simulink model "Weiv_filter_V1_1"  (R2017b)
settings: Solver=ode4  StartTime=0.0  StopTime=5.9443  RelTol=1e-3
undefined symbols (not defined in the file or in its folder): dfilt, get
libraries: dspobslib x2, dspvision x1, dspsnks4 x1
settings Model: Creator=root  LastModifiedBy=root

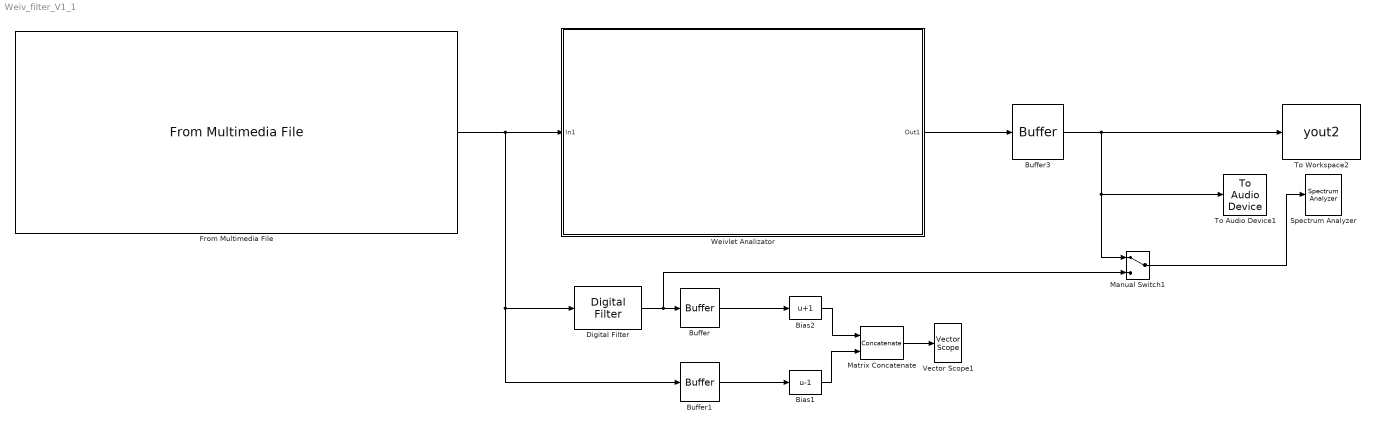
== system Weiv_filter_V1_1 ==
  Bias1 : Bias  Bias=-1
  Bias2 : Bias  Bias=1
  Buffer : Buffer  N=441
  Buffer1 : Buffer  N=441
  Buffer3 : Buffer  N=512
  Digital Filter : dspobslib/Digital Filter  TypePopup=IIR (poles & zeros)  IIRFiltStruct=Direct form II transposed  AllPoleFiltStruct=Direct form  FIRFiltStruct=Direct form  CoeffSource=Specify via dialog  NumCoeffs=[0 0.0554]  DenCoeffs=[1 -0.9446]  BiQuadCoeffs=[1 0.3 0.4 1 0.1 0.2]  LatticeCoeffs=[0.2 0.4]  denIgnore=on  FiltPerSampPopup=One filter per frame  IC=0  ICnum=0  ICden=0  roundingMode=Floor  overflowMode=off  ScaleValues=1  scaleValueFracLength=14  stageInFracLength=15  stageOutFracLength=15  FilterSource=Specify via dialog  dfiltObjectName=dfilt.dffir([1 2 1])  InputProcessing=Inherited (this choice will be removed - see release notes)
      settings: SourceProductName=DSP System Toolbox  SourceProductBaseCode=DS
  From Multimedia File : dspvision/From Multimedia File  inputFilename=/mnt/work/develop/matlab/voip/source/58691/MyTest.wav  loop=on  numPlays=inf  outputStreams=Audio only  videoDataType=single  audioDataType=double  inheritSampleTime=on  userDefinedSampleTime=1/30  noAudioOutput=off  isIntensityVideo=off  fourcc=RGB  colorVideoFormat=Separate color signals  outputEOF=off  dataOrg=Column-major  audioFrameSize=512  computeAudioFrameSize=off  outSamplingMode=Frame based
      settings: SourceProductBaseCode=VP
  Manual Switch1 : ManualSwitch
  Matrix Concatenate : Concatenate  Mode=Multidimensional array  ConcatenateDimension=2
  Spectrum Analyzer : SpectrumAnalyzer
  To Audio Device1 : dspobslib/To Audio Device  deviceName=Default  inheritSampleRate=on  sampleRate=44100  deviceDatatype=Determine from input data type  autoBufferSize=on  bufferSize=4096  queueDuration=1.0  defaultOutputChannelMapping=on  outputChannelMapping=1:2  outputNumUnderrunSamples=off
      settings: SourceProductName=DSP System Toolbox  SourceProductBaseCode=DS
  To Workspace2 : ToWorkspace  VariableName=yout2  SaveFormat=Structure  SampleTime=-1
      settings: Save2DSignal=2-D array (concatenate along first dimension)
  Vector Scope1 : dspsnks4/Vector Scope  ScopeProperties=on  Domain=Time  HorizSpan=1  DisplayProperties=off  AxisGrid=on  Memory=off  FrameNumber=on  AxisLegend=off  AxisZoom=off  OpenScopeAtSimStart=on  OpenScopeImmediately=off  FigPos=get(0,'defaultfigureposition')  AxisProperties=off  XUnits=Hertz  XRange=[0...Fs/2]  InheritXIncr=on  XIncr=1  XLabel=Time  XLimit=Auto  XMin=-0.001  XMax=0.001  XStart=0  YUnits=dB  YLabel=Amplitude  LineProperties=off  LineColors='k' | 'r'  XAxisParamsVer=6.9
      settings: SourceProductName=DSP System Toolbox  SourceProductBaseCode=DS  YMin=-2  YMax=2
  Weivlet Analizator : Subsystem
  wires:
  From Multimedia File/1 -> Buffer1/1, Digital Filter/1, Weivlet Analizator/1(In1)
  Bias1/1 -> Matrix Concatenate/2
  Buffer/1 -> Bias2/1
  Matrix Concatenate/1 -> Vector Scope1/1
  Buffer1/1 -> Bias1/1
  Bias2/1 -> Matrix Concatenate/1
  Buffer3/1 -> To Workspace2/1, Manual Switch1/1, To Audio Device1/1
  Digital Filter/1 -> Manual Switch1/2, Buffer/1
  Manual Switch1/1 -> Spectrum Analyzer/1
  Weivlet Analizator/1(Out1) -> Buffer3/1

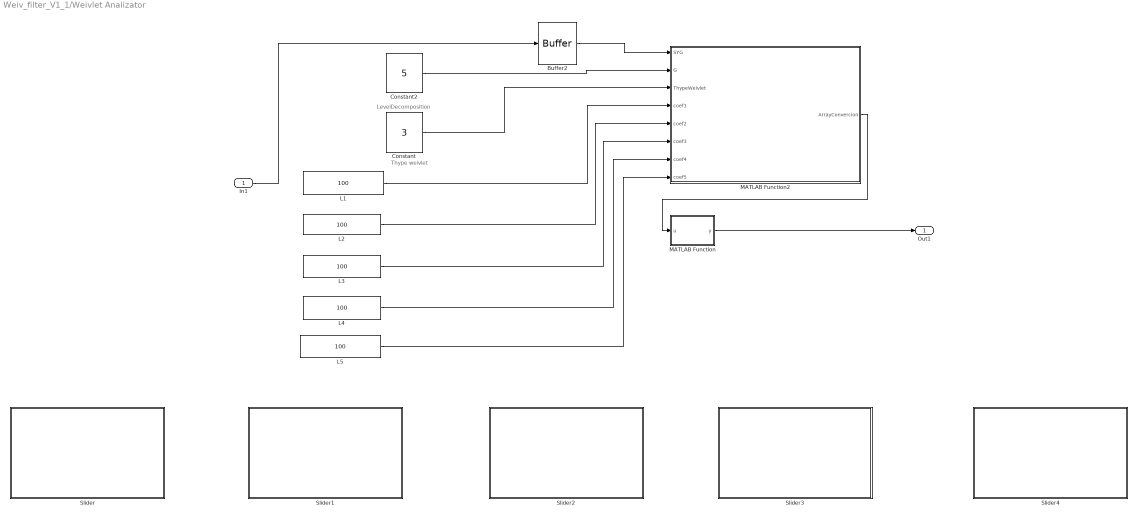
== system Weiv_filter_V1_1/Weivlet Analizator ==
  note: Thype weivlet
  note: LevelDecomposition
  In1 : Inport
  Buffer2 : Buffer  N=512
  Constant : Constant  Value=3
  Constant2 : Constant  Value=5
  L{1..5} (5 alike) : Constant  Value=100
  MATLAB Function : MATLAB Function  TreatAsAtomicUnit=on
  MATLAB Function2 : MATLAB Function  TreatAsAtomicUnit=on
  Slider : Subsystem  DialogController=hmiCreateDDGDialog  IsWebBlock=on  mask(MWDashboardBlock){webBlockId=768a49ab-0276-4495-b760-370aa239fe65, webBlockType=slider, ShowInLibBrowser=on, ShowInitialText=on, HMISrcModelName=Test}
      mask prompts: webBlockId "WebBlock Id"; webBlockType "WebBlock Type"; HMISrcModelName "Source Model"
      mask help: SimulinkHMI:dialogs:SliderDialogDesc
      mask Help: helpview([docroot '/mapfiles/simulink.map'], 'hmi_slider')
      mask Display:
      | if strcmp(get_param(bdroot(gcb),'BlockDiagramType'), 'library')
      |     image([(matlabroot) '/toolbox/simulink/hmi/icons/Slider.png']);
      | end
  Slider1 : Subsystem  DialogController=hmiCreateDDGDialog  IsWebBlock=on  mask(MWDashboardBlock){webBlockId=323077e0-7fcc-417c-936f-3810df4c105c, webBlockType=slider, ShowInLibBrowser=on, ShowInitialText=on, HMISrcModelName=Test}
      mask prompts: webBlockId "WebBlock Id"; webBlockType "WebBlock Type"; HMISrcModelName "Source Model"
      mask help: SimulinkHMI:dialogs:SliderDialogDesc
      mask Help: helpview([docroot '/mapfiles/simulink.map'], 'hmi_slider')
      mask Display:
      | if strcmp(get_param(bdroot(gcb),'BlockDiagramType'), 'library')
      |     image([(matlabroot) '/toolbox/simulink/hmi/icons/Slider.png']);
      | end
  Slider2 : Subsystem  DialogController=hmiCreateDDGDialog  IsWebBlock=on  mask(MWDashboardBlock){webBlockId=d4f9fa27-d2d0-4c83-acb2-83c8f6e37425, webBlockType=slider, ShowInLibBrowser=on, ShowInitialText=on, HMISrcModelName=Test}
      mask prompts: webBlockId "WebBlock Id"; webBlockType "WebBlock Type"; HMISrcModelName "Source Model"
      mask help: SimulinkHMI:dialogs:SliderDialogDesc
      mask Help: helpview([docroot '/mapfiles/simulink.map'], 'hmi_slider')
      mask Display:
      | if strcmp(get_param(bdroot(gcb),'BlockDiagramType'), 'library')
      |     image([(matlabroot) '/toolbox/simulink/hmi/icons/Slider.png']);
      | end
  Slider3 : Subsystem  DialogController=hmiCreateDDGDialog  IsWebBlock=on  mask(MWDashboardBlock){webBlockId=c3419087-b37d-482c-b4cc-896f47945971, webBlockType=slider, ShowInLibBrowser=on, ShowInitialText=on, HMISrcModelName=Test}
      mask prompts: webBlockId "WebBlock Id"; webBlockType "WebBlock Type"; HMISrcModelName "Source Model"
      mask help: SimulinkHMI:dialogs:SliderDialogDesc
      mask Help: helpview([docroot '/mapfiles/simulink.map'], 'hmi_slider')
      mask Display:
      | if strcmp(get_param(bdroot(gcb),'BlockDiagramType'), 'library')
      |     image([(matlabroot) '/toolbox/simulink/hmi/icons/Slider.png']);
      | end
  Slider4 : Subsystem  DialogController=hmiCreateDDGDialog  IsWebBlock=on  mask(MWDashboardBlock){webBlockId=d8735f17-68f6-4fd6-86dc-e3ad28bdaaeb, webBlockType=slider, ShowInLibBrowser=on, ShowInitialText=on, HMISrcModelName=Test}
      mask prompts: webBlockId "WebBlock Id"; webBlockType "WebBlock Type"; HMISrcModelName "Source Model"
      mask help: SimulinkHMI:dialogs:SliderDialogDesc
      mask Help: helpview([docroot '/mapfiles/simulink.map'], 'hmi_slider')
      mask Display:
      | if strcmp(get_param(bdroot(gcb),'BlockDiagramType'), 'library')
      |     image([(matlabroot) '/toolbox/simulink/hmi/icons/Slider.png']);
      | end
  Out1 : Outport
  wires:
  In1/1 -> Buffer2/1
  Constant2/1 -> MATLAB Function2/2(G)
  Constant/1 -> MATLAB Function2/3(ThypeWeivlet)
  Buffer2/1 -> MATLAB Function2/1(SYG)
  MATLAB Function2/1(ArrayConvercion) -> MATLAB Function/1(u)
  MATLAB Function/1(y) -> Out1/1
  L5/1 -> MATLAB Function2/8(coef5)
  L4/1 -> MATLAB Function2/7(coef4)
  L3/1 -> MATLAB Function2/6(coef3)
  L2/1 -> MATLAB Function2/5(coef2)
  L1/1 -> MATLAB Function2/4(coef1)

== system Weiv_filter_V1_1/Weivlet Analizator/Slider ==

== system Weiv_filter_V1_1/Weivlet Analizator/Slider1 ==

== system Weiv_filter_V1_1/Weivlet Analizator/Slider2 ==

== system Weiv_filter_V1_1/Weivlet Analizator/Slider3 ==

== system Weiv_filter_V1_1/Weivlet Analizator/Slider4 ==

== matlab function Weiv_filter_V1_1/Weivlet Analizator/MATLAB Function ==
  data: u input double size=[585,1] [0..585]; y output
function y = costil(u)
y=zeros(512,1,'double');
            u=u(:);
            coder.varsize('u', [585 1]); 
        if length(u)< 585

            y = u(1:512);
        end
            
%         elseif length(u)< 1083
%             
%             y=zeros(1084,1,'double');
%             
%         end
end

% y = u;

== matlab function Weiv_filter_V1_1/Weivlet Analizator/MATLAB Function2 ==
  settings: sampleTime=1
  data: SYG input double; G input double; ThypeWeivlet input double; ArrayConvercion output double size=[585,1] [0..585]; coef1 input; coef2 input; coef3 input; coef4 input; coef5 input
function ArrayConvercion = DirectWaivletSimilink(SYG,G,ThypeWeivlet,coef1,coef2,coef3,coef4,coef5)
% direct wavelet conversion
%Autor Starokoszev S.V. 26.02.18
structweiv={'haar','db1','sym8'};
Thype=structweiv{1,ThypeWeivlet};
coder.extrinsic('wfilters'); 
coder.extrinsic('wavedec'); 
coder.extrinsic('waverec');
coder.extrinsic('wmaxlev'); 

NumbComponent=G;
Y1=SYG;
N=G;
[Lo_D,Hi_D] = wfilters(Thype,'d');%filter for decomposition 
C=zeros(585,1);
% [C L1] = wavedec(SYG,5,Lo_D,Hi_D);

[Lo_R,Hi_R] = wfilters(Thype,'r');

N = wmaxlev(length(Y1),'sym8');
[C L1]=wavedec(Y1,N,'sym8');
% coef1=100;
% coef2=100;
% coef3=100;
% coef4=100;
% coef5=100;
mass_coef=zeros(1,N,'double');
mass_coef(1)=coef5;
mass_coef(2)=coef4;
mass_coef(3)=coef3;
mass_coef(4)=coef2;
mass_coef(5)=coef1;
en=0;
t1=1;
t1=double(t1);
en=length(L1);
L_new=zeros(5,1,'double');
L_new=L1(2:en-1);
idx=0;
% endn=zeros(1,length(L_new),'double');
endn=zeros(1,5,'double');
endn=double(endn);
% idx=double(idx);
idx=N;
 OutputArray=zeros(585,1,'double');
 l_new_idx=1;
  start=0;
  gg=0;
  
  
while idx >=1 
    
%     cd_N=detcoef(C,L1,idx);
    if idx==N
            tmp=(C(1:L_new(t1)).*mass_coef(N))./100;
            for i=1:1:L_new(t1)
                OutputArray(i)=tmp(i);
            end
            for i=L_new(t1):1:(L_new(t1)+L_new(t1))
            OutputArray(i)=(C(i)*mass_coef(N))/100;
            end
    end
if idx < N
    start=L_new(t1);
    gg=0;
                for sum_ind=1:1:l_new_idx
                start=start + L_new(sum_ind); 
                endn(sum_ind)=start;
               gg=gg+1;
                end
    str = endn(gg-1);
    endn1= endn(gg);

                 for i= str:1:endn1
                       OutputArray(i) = (C(i)*mass_coef(idx))/100;
                 end
end
l_new_idx=l_new_idx+1;
idx=idx-1;
end
ArrayConvercion=waverec(OutputArray,L1,Lo_D,Hi_D);
end
